simulink model "OCR"  (Simulink 10.0)
settings: Solver=ode23tb  StartTime=0.0  StopTime=10  RelTol=1e-3  EnableMultiTasking=on
libraries: powerlib x36, powerlib_extras x12, simulink x6
settings Model: Creator=Khan  LastModifiedBy=bhisma
settings DataIOCC: LimitDataPoints=on  SignalLoggingSaveFormat=ModelDataLogs
settings OptimizationCC: ExpressionDepthLimit=2147483647  InitFltsAndDblsToZero=on
settings DebuggingCC: SaveWithParameterizedLinksMsg=none  SignalResolutionControl=TryResolveAllWithWarning  MultiTaskDSMMsg=warning  MultiTaskCondExecSysMsg=none  FcnCallInpInsideContextMsg=warning  StateNameClashWarn=warning
settings SFSimCC: SimParseCustomCode=off
settings GRTTargetCC: TargetFcnLib=ansi_tfl_tmw.mat  GeneratePreprocessorConditionals=Disable all
settings ConfigComp: CovExternalEMLEnable=off

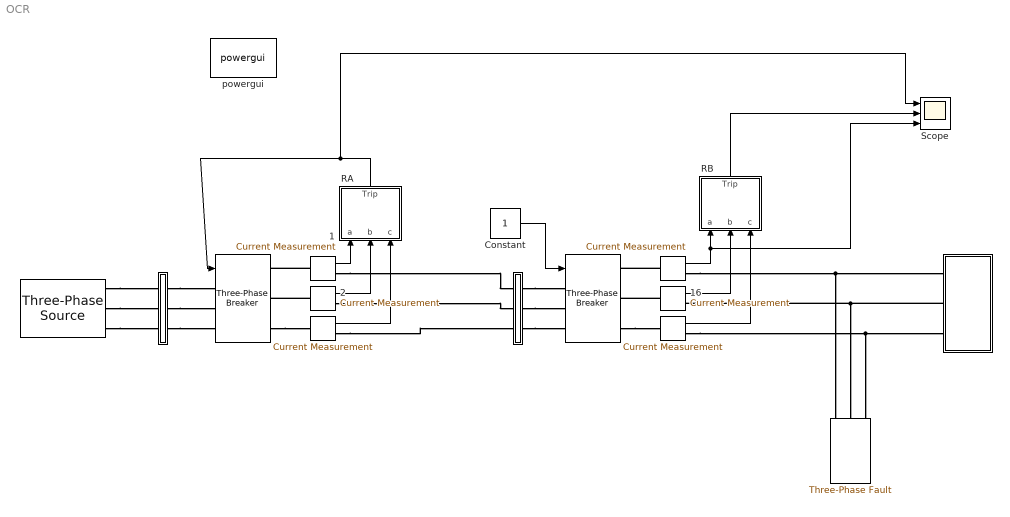
== system OCR ==
  "     " : powerlib/Measurements/Current Measurement  SystemSampleTime=-1  PhasorSimulation=off  OutputType=Complex  PSBequivalent=0
      settings: SourceProductName=Simscape Electrical
  "                                                     " : powerlib/Measurements/Current Measurement  SystemSampleTime=-1  PhasorSimulation=off  OutputType=Complex  PSBequivalent=0
      settings: SourceProductName=Simscape Electrical
  "                                                            " : powerlib/Measurements/Current Measurement  SystemSampleTime=-1  PhasorSimulation=off  OutputType=Complex  PSBequivalent=0
      settings: SourceProductName=Simscape Electrical
  " 1" : powerlib/Measurements/Current Measurement  SystemSampleTime=-1  PhasorSimulation=off  OutputType=Complex  PSBequivalent=0
      settings: SourceProductName=Simscape Electrical
  " 16" : powerlib/Measurements/Current Measurement  SystemSampleTime=-1  PhasorSimulation=off  OutputType=Complex  PSBequivalent=0
      settings: SourceProductName=Simscape Electrical
  " 2" : powerlib/Measurements/Current Measurement  SystemSampleTime=-1  PhasorSimulation=off  OutputType=Complex  PSBequivalent=0
      settings: SourceProductName=Simscape Electrical
  " " : powerlib/Elements/Three-Phase Breaker  SystemSampleTime=-1  InitialState=closed  SwitchA=on  SwitchB=on  SwitchC=on  SwitchTimes=1000000000  External=on  BreakerResistance=0.001  SnubberResistance=1e6  SnubberCapacitance=inf  Measurements=None
      link override Breaker A: Measurements=None
      link override Breaker B: Measurements=None
      link override Breaker C: Measurements=None
      settings: SourceProductName=Simscape Electrical
  "    " : Subsystem
      mask Display: disp('')
  "      " : powerlib/Elements/Three-Phase Breaker  SystemSampleTime=-1  InitialState=closed  SwitchA=on  SwitchB=on  SwitchC=on  SwitchTimes=1000000000  External=on  BreakerResistance=0.001  SnubberResistance=1e6  SnubberCapacitance=inf  Measurements=None
      link override Breaker A: Measurements=None
      link override Breaker B: Measurements=None
      link override Breaker C: Measurements=None
      settings: SourceProductName=Simscape Electrical
  "       " : Subsystem
      mask Display: disp('')
  "               " : powerlib/Elements/Three-Phase Fault  SystemSampleTime=-1  FaultA=on  FaultB=on  FaultC=on  FaultResistance=0.6  GroundFault=on  GroundResistance=1000000  External=off  SwitchStatus=[1]  SwitchTimes=[ 6]  InitialStates=[0 0 1]  SnubberResistance=1e6  SnubberCapacitance=inf  Measurements=None
      settings: SourceProductName=Simscape Electrical
  "                            " : Subsystem
  "                                           " : powerlib/Electrical Sources/Three-Phase Source  SystemSampleTime=-1  Voltage=400  PhaseAngle=0  Frequency=50  InternalConnection=Yg  SpecifyImpedance=on  Resistance=25^2/1000/10  Inductance=25^2/1000/377  ShortCircuitLevel=1020e6  BaseVoltage=400  XRratio=10
      settings: SourceProductName=Simscape Electrical
  Constant : Constant
  RA : Subsystem
  RB : Subsystem
  Scope : Scope  NumInputPorts=3
  powergui : powerlib/powergui  Priority=1  SystemSampleTime=-1  SimulationMode=Continuous  SampleTime=50e-6  frequency=60  SPID=off  DisableSnubberDevices=off  DisableRonSwitches=off  DisableVfSwitches=off  SwTol=0  Interpol=off  frequencyindice=0  echomessages=off  HookPort=off  DisplayEquations=off  FunctionMessages=off  EnableUseOfTLC=off  x0status=blocks  RestoreLinks=warning  ResistiveCurrentMeasurement=off  Ylog=off  Xlog=on  ShowGrid=off  save=off  variable=ZData  ZoomFFT=off  StartTime=0.0  cycles=1  DisplayStyle=1  FreqAxis=off  MaxFrequency=1000  frequencyindicesteady=1  display=off  methode=off
      settings: SourceProductName=Simscape Electrical
  wires:
  "                                                            "/1 -> Scope/3, RB/1(a)
  " 16"/1 -> RB/2(b)
  "                                                     "/1 -> RB/3(c)
  RB/1(Trip) -> Scope/2
  " 1"/1 -> RA/1(a)
  " 2"/1 -> RA/2(b)
  "     "/1 -> RA/3(c)
  RA/1(Trip) -> "      "/1, Scope/1
  Constant/1 -> " "/1
  connections:
  "                                                            "/LConn1 -- " "/RConn1
  " 16"/LConn1 -- " "/RConn2
  " "/RConn3 -- "                                                     "/LConn1
  "                                                            "/RConn1 -- "                            "/LConn1 -- "               "/LConn1
  "                            "/LConn2 -- " 16"/RConn1 -- "               "/LConn2
  "                                                     "/RConn1 -- "                            "/LConn3 -- "               "/LConn3
  " 2"/LConn1 -- "      "/RConn2
  " 1"/LConn1 -- "      "/RConn1
  "      "/RConn3 -- "     "/LConn1
  "    "/RConn3 -- " "/LConn3
  "    "/RConn2 -- " "/LConn2
  "    "/RConn1 -- " "/LConn1
  " 1"/RConn1 -- "    "/LConn1
  " 2"/RConn1 -- "    "/LConn2
  "     "/RConn1 -- "    "/LConn3
  "                                           "/RConn3 -- "       "/RConn3
  "                                           "/RConn2 -- "       "/RConn2
  "                                           "/RConn1 -- "       "/RConn1
  "       "/LConn3 -- "      "/LConn3
  "       "/LConn2 -- "      "/LConn2
  "       "/LConn1 -- "      "/LConn1

== system OCR/     ==
  A1 : PMIOPort  Side=Left
  B1 : PMIOPort  Port=2  Side=Left
  C1 : PMIOPort  Port=3  Side=Left
  A2 : PMIOPort  Port=4  Side=Right
  B2 : PMIOPort  Port=5  Side=Right
  C2 : PMIOPort  Port=6  Side=Right
  connections:
  C1/RConn1 -- C2/RConn1
  B1/RConn1 -- B2/RConn1
  A1/RConn1 -- A2/RConn1

== system OCR/        ==
  A1 : PMIOPort  Side=Left
  B1 : PMIOPort  Port=2  Side=Left
  C1 : PMIOPort  Port=3  Side=Left
  A2 : PMIOPort  Port=4  Side=Right
  B2 : PMIOPort  Port=5  Side=Right
  C2 : PMIOPort  Port=6  Side=Right
  connections:
  A1/RConn1 -- A2/RConn1
  B1/RConn1 -- B2/RConn1
  C1/RConn1 -- C2/RConn1

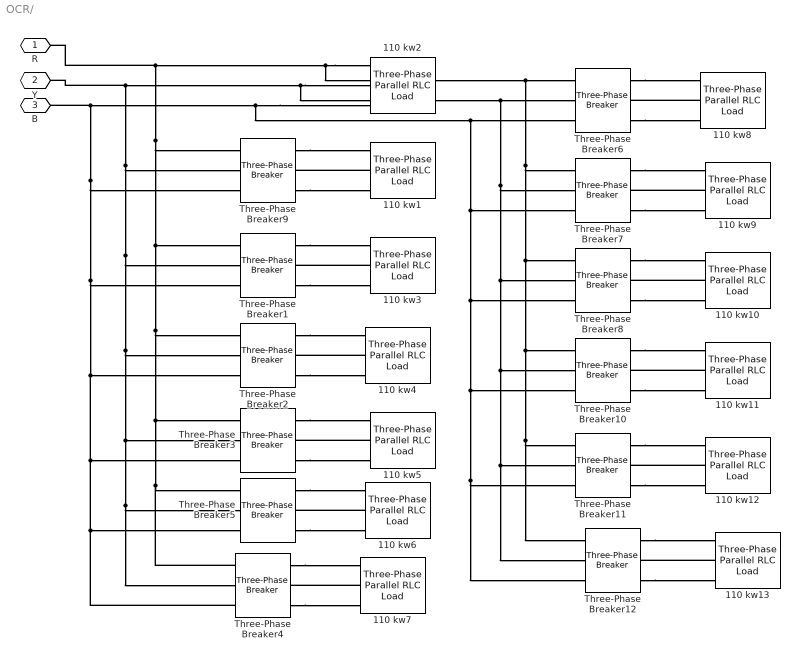
== system OCR/                             ==
  110 kw{1,3..13} (12 alike) : powerlib/Elements/Three-Phase Parallel RLC Load  PhysicalDomain=powersysdomain  SubClassName=unknown  LeftPortType=p1  RightPortType=p1  LConnTagsString=A|B|C  Configuration=Y (grounded)  NominalVoltage=400  NominalFrequency=50  ActivePower=110e3/4  InductivePower=58e3/4  CapacitivePower=0  Measurements=None
      settings: SourceProductName=Simscape Electrical
  110 kw2 : powerlib/Elements/Three-Phase Parallel RLC Load  PhysicalDomain=powersysdomain  SubClassName=unknown  LeftPortType=p1  RightPortType=p1  LConnTagsString=A|B|C  Configuration=Y (grounded)  NominalVoltage=400  NominalFrequency=50  ActivePower=110e3  InductivePower=58e3  CapacitivePower=0  Measurements=None
      settings: SourceProductName=Simscape Electrical
  Three-Phase Breaker1 : powerlib/Elements/Three-Phase Breaker  SystemSampleTime=-1  InitialState=closed  SwitchA=on  SwitchB=on  SwitchC=on  SwitchTimes=1.25  External=off  BreakerResistance=0.001  SnubberResistance=1e6  SnubberCapacitance=inf  Measurements=None
      settings: SourceProductName=Simscape Electrical
  Three-Phase Breaker10 : powerlib/Elements/Three-Phase Breaker  SystemSampleTime=-1  InitialState=closed  SwitchA=on  SwitchB=on  SwitchC=on  SwitchTimes=2.25  External=off  BreakerResistance=0.001  SnubberResistance=1e6  SnubberCapacitance=inf  Measurements=None
      settings: SourceProductName=Simscape Electrical
  Three-Phase Breaker11 : powerlib/Elements/Three-Phase Breaker  SystemSampleTime=-1  InitialState=closed  SwitchA=on  SwitchB=on  SwitchC=on  SwitchTimes=2  External=off  BreakerResistance=0.001  SnubberResistance=1e6  SnubberCapacitance=inf  Measurements=None
      settings: SourceProductName=Simscape Electrical
  Three-Phase Breaker12 : powerlib/Elements/Three-Phase Breaker  SystemSampleTime=-1  InitialState=closed  SwitchA=on  SwitchB=on  SwitchC=on  SwitchTimes=1.75  External=off  BreakerResistance=0.001  SnubberResistance=1e6  SnubberCapacitance=inf  Measurements=None
      settings: SourceProductName=Simscape Electrical
  Three-Phase Breaker2 : powerlib/Elements/Three-Phase Breaker  SystemSampleTime=-1  InitialState=closed  SwitchA=on  SwitchB=on  SwitchC=on  SwitchTimes=1  External=off  BreakerResistance=0.001  SnubberResistance=1e6  SnubberCapacitance=inf  Measurements=None
      settings: SourceProductName=Simscape Electrical
  Three-Phase Breaker3 : powerlib/Elements/Three-Phase Breaker  SystemSampleTime=-1  InitialState=closed  SwitchA=on  SwitchB=on  SwitchC=on  SwitchTimes=0.75  External=off  BreakerResistance=0.001  SnubberResistance=1e6  SnubberCapacitance=inf  Measurements=None
      settings: SourceProductName=Simscape Electrical
  Three-Phase Breaker4 : powerlib/Elements/Three-Phase Breaker  SystemSampleTime=-1  InitialState=closed  SwitchA=on  SwitchB=on  SwitchC=on  SwitchTimes=0.25  External=off  BreakerResistance=0.001  SnubberResistance=1e6  SnubberCapacitance=inf  Measurements=None
      settings: SourceProductName=Simscape Electrical
  Three-Phase Breaker5 : powerlib/Elements/Three-Phase Breaker  SystemSampleTime=-1  InitialState=closed  SwitchA=on  SwitchB=on  SwitchC=on  SwitchTimes=0.5  External=off  BreakerResistance=0.001  SnubberResistance=1e6  SnubberCapacitance=inf  Measurements=None
      settings: SourceProductName=Simscape Electrical
  Three-Phase Breaker6 : powerlib/Elements/Three-Phase Breaker  SystemSampleTime=-1  InitialState=closed  SwitchA=on  SwitchB=on  SwitchC=on  SwitchTimes=3  External=off  BreakerResistance=0.001  SnubberResistance=1e6  SnubberCapacitance=inf  Measurements=None
      settings: SourceProductName=Simscape Electrical
  Three-Phase Breaker7 : powerlib/Elements/Three-Phase Breaker  SystemSampleTime=-1  InitialState=closed  SwitchA=on  SwitchB=on  SwitchC=on  SwitchTimes=2.75  External=off  BreakerResistance=0.001  SnubberResistance=1e6  SnubberCapacitance=inf  Measurements=None
      settings: SourceProductName=Simscape Electrical
  Three-Phase Breaker8 : powerlib/Elements/Three-Phase Breaker  SystemSampleTime=-1  InitialState=closed  SwitchA=on  SwitchB=on  SwitchC=on  SwitchTimes=2.5  External=off  BreakerResistance=0.001  SnubberResistance=1e6  SnubberCapacitance=inf  Measurements=None
      settings: SourceProductName=Simscape Electrical
  Three-Phase Breaker9 : powerlib/Elements/Three-Phase Breaker  SystemSampleTime=-1  InitialState=closed  SwitchA=on  SwitchB=on  SwitchC=on  SwitchTimes=1.5  External=off  BreakerResistance=0.001  SnubberResistance=1e6  SnubberCapacitance=inf  Measurements=None
      settings: SourceProductName=Simscape Electrical
  " R" : PMIOPort  Side=Left
  "Y " : PMIOPort  Port=2  Side=Left
  "B   " : PMIOPort  Port=3  Side=Left
  connections:
  Three-Phase Breaker3/LConn1 -- Three-Phase Breaker4/LConn1 -- Three-Phase Breaker5/LConn1 -- Three-Phase Breaker2/LConn1 -- Three-Phase Breaker1/LConn1 -- Three-Phase Breaker9/LConn1 -- " R"/RConn1 -- 110 kw2/LConn1 -- Three-Phase Breaker6/LConn1 -- Three-Phase Breaker7/LConn1 -- Three-Phase Breaker8/LConn1 -- Three-Phase Breaker10/LConn1 -- Three-Phase Breaker11/LConn1 -- Three-Phase Breaker12/LConn1
  Three-Phase Breaker3/LConn2 -- Three-Phase Breaker4/LConn2 -- Three-Phase Breaker5/LConn2 -- Three-Phase Breaker2/LConn2 -- Three-Phase Breaker1/LConn2 -- Three-Phase Breaker9/LConn2 -- "Y "/RConn1 -- 110 kw2/LConn2 -- Three-Phase Breaker6/LConn2 -- Three-Phase Breaker7/LConn2 -- Three-Phase Breaker8/LConn2 -- Three-Phase Breaker10/LConn2 -- Three-Phase Breaker12/LConn2 -- Three-Phase Breaker11/LConn2
  "B   "/RConn1 -- Three-Phase Breaker12/LConn3 -- Three-Phase Breaker11/LConn3 -- Three-Phase Breaker10/LConn3 -- Three-Phase Breaker8/LConn3 -- Three-Phase Breaker7/LConn3 -- Three-Phase Breaker6/LConn3 -- 110 kw2/LConn3 -- Three-Phase Breaker2/LConn3 -- Three-Phase Breaker3/LConn3 -- Three-Phase Breaker4/LConn3 -- Three-Phase Breaker5/LConn3 -- Three-Phase Breaker1/LConn3 -- Three-Phase Breaker9/LConn3
  Three-Phase Breaker9/RConn1 -- 110 kw1/LConn1
  110 kw1/LConn2 -- Three-Phase Breaker9/RConn2
  Three-Phase Breaker9/RConn3 -- 110 kw1/LConn3
  Three-Phase Breaker1/RConn3 -- 110 kw3/LConn3
  110 kw3/LConn2 -- Three-Phase Breaker1/RConn2
  Three-Phase Breaker1/RConn1 -- 110 kw3/LConn1
  Three-Phase Breaker2/RConn1 -- 110 kw4/LConn1
  110 kw4/LConn2 -- Three-Phase Breaker2/RConn2
  Three-Phase Breaker2/RConn3 -- 110 kw4/LConn3
  Three-Phase Breaker3/RConn3 -- 110 kw5/LConn3
  110 kw5/LConn2 -- Three-Phase Breaker3/RConn2
  Three-Phase Breaker3/RConn1 -- 110 kw5/LConn1
  Three-Phase Breaker4/RConn1 -- 110 kw7/LConn1
  110 kw7/LConn2 -- Three-Phase Breaker4/RConn2
  Three-Phase Breaker4/RConn3 -- 110 kw7/LConn3
  Three-Phase Breaker5/RConn1 -- 110 kw6/LConn1
  110 kw6/LConn2 -- Three-Phase Breaker5/RConn2
  Three-Phase Breaker5/RConn3 -- 110 kw6/LConn3
  Three-Phase Breaker6/RConn3 -- 110 kw8/LConn3
  110 kw8/LConn2 -- Three-Phase Breaker6/RConn2
  Three-Phase Breaker6/RConn1 -- 110 kw8/LConn1
  Three-Phase Breaker7/RConn1 -- 110 kw9/LConn1
  110 kw9/LConn2 -- Three-Phase Breaker7/RConn2
  Three-Phase Breaker7/RConn3 -- 110 kw9/LConn3
  Three-Phase Breaker8/RConn3 -- 110 kw10/LConn3
  Three-Phase Breaker8/RConn1 -- 110 kw10/LConn1
  110 kw10/LConn2 -- Three-Phase Breaker8/RConn2
  110 kw11/LConn2 -- Three-Phase Breaker10/RConn2
  Three-Phase Breaker10/RConn1 -- 110 kw11/LConn1
  Three-Phase Breaker10/RConn3 -- 110 kw11/LConn3
  Three-Phase Breaker11/RConn3 -- 110 kw12/LConn3
  Three-Phase Breaker11/RConn1 -- 110 kw12/LConn1
  110 kw12/LConn2 -- Three-Phase Breaker11/RConn2
  110 kw13/LConn2 -- Three-Phase Breaker12/RConn2
  Three-Phase Breaker12/RConn3 -- 110 kw13/LConn3
  Three-Phase Breaker12/RConn1 -- 110 kw13/LConn1

== system OCR/RA ==
  a : Inport
  b : Inport  Port=2
  c : Inport  Port=3
  " 18" : DataTypeConversion  OutDataTypeStr=double
  Logical Operator : Logic  Inputs=3  AllPortsSameDT=off  OutDataTypeStr=boolean
  phase a : Subsystem
  phase a1 : Subsystem
  phase a2 : Subsystem
  Trip : Outport
  wires:
  " 18"/1 -> Trip/1
  c/1 -> phase a2/1(In1)
  b/1 -> phase a1/1(In1)
  a/1 -> phase a/1(In1)
  phase a/1(Out1) -> Logical Operator/1
  Logical Operator/1 -> " 18"/1
  phase a2/1(Out1) -> Logical Operator/3
  phase a1/1(Out1) -> Logical Operator/2

== system OCR/RB ==
  a : Inport
  b : Inport  Port=2
  c : Inport  Port=3
  " 18" : DataTypeConversion  OutDataTypeStr=double
  Logical Operator : Logic  Inputs=3  AllPortsSameDT=off  OutDataTypeStr=boolean
  phase a : Subsystem
  phase a1 : Subsystem
  phase a2 : Subsystem
  Trip : Outport
  wires:
  phase a1/1(Out1) -> Logical Operator/2
  phase a2/1(Out1) -> Logical Operator/3
  Logical Operator/1 -> " 18"/1
  phase a/1(Out1) -> Logical Operator/1
  a/1 -> phase a/1(In1)
  b/1 -> phase a1/1(In1)
  c/1 -> phase a2/1(In1)
  " 18"/1 -> Trip/1

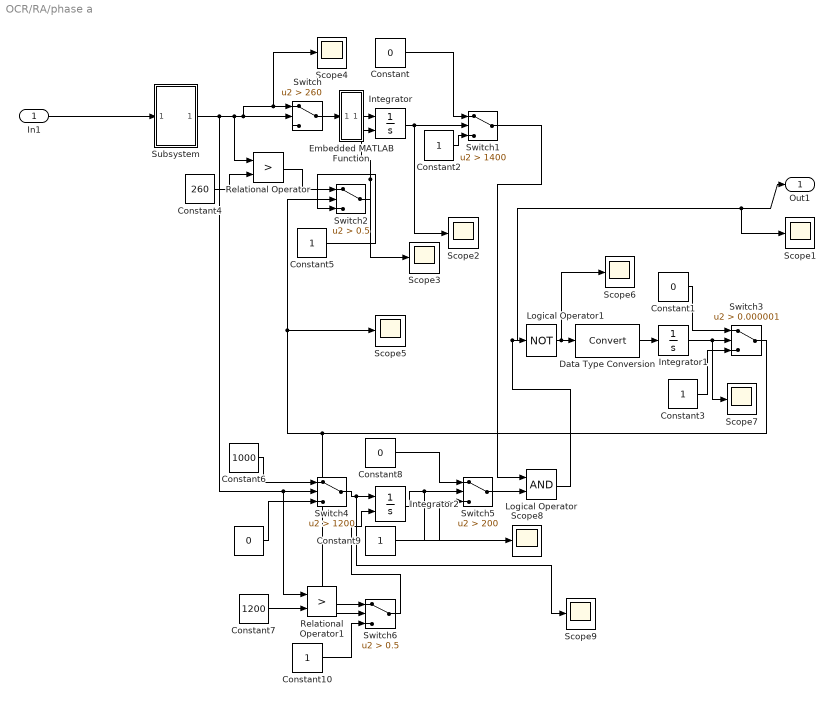
== system OCR/RA/phase a ==
  In1 : Inport
  " " : Constant  Value=0
  Constant : Constant  Value=0
  Constant1 : Constant  Value=0
  Constant{2..3,5,9..10} (5 alike) : Constant
  Constant4 : Constant  Value=260
  Constant6 : Constant  Value=1000
  Constant7 : Constant  Value=1200
  Constant8 : Constant  Value=0
  Data Type Conversion : DataTypeConversion
  Embedded MATLAB Function : MATLAB Function  TreatAsAtomicUnit=on
  Integrator : Integrator  ExternalReset=falling
  Integrator1 : Integrator
  Integrator2 : Integrator  ExternalReset=falling
  Logical Operator : Logic  AllPortsSameDT=off  OutDataTypeStr=boolean
  Logical Operator1 : Logic  Operator=NOT  AllPortsSameDT=off  OutDataTypeStr=boolean
  Relational Operator : RelationalOperator  Operator=>  OutDataTypeStr=boolean  RndMeth=Nearest
  Relational Operator1 : RelationalOperator  Operator=>  OutDataTypeStr=boolean  RndMeth=Nearest
  Scope{1..9} (9 alike) : Scope
  Subsystem : Subsystem
  Switch : Switch  Criteria=u2 > Threshold  Threshold=260
  Switch1 : Switch  Criteria=u2 > Threshold  Threshold=1400  ZeroCross=off
  Switch2 : Switch  Criteria=u2 > Threshold  Threshold=0.5
  Switch3 : Switch  Criteria=u2 > Threshold  Threshold=0.000001
  Switch4 : Switch  Criteria=u2 > Threshold  Threshold=1200
  Switch5 : Switch  Criteria=u2 > Threshold  Threshold=200  ZeroCross=off
  Switch6 : Switch  Criteria=u2 > Threshold  Threshold=0.5
  Out1 : Outport
  wires:
  Switch6/1 -> Integrator2/2
  Constant10/1 -> Switch6/3
  Relational Operator1/1 -> Switch6/1
  Constant7/1 -> Relational Operator1/2
  Logical Operator/1 -> Scope1/1, Out1/1, Logical Operator1/1
  Switch5/1 -> Logical Operator/2
  Constant9/1 -> Switch5/3
  Constant8/1 -> Switch5/1
  Integrator2/1 -> Scope8/1, Switch5/2
  Switch4/1 -> Scope9/1, Integrator2/1
  " "/1 -> Switch4/3
  Constant6/1 -> Switch4/1
  Embedded MATLAB Function/1(y) -> Integrator/1
  Switch3/1 -> Switch6/2, Scope5/1, Switch2/2
  Constant1/1 -> Switch3/1
  Integrator1/1 -> Switch3/2, Scope7/1
  Data Type Conversion/1 -> Integrator1/1
  Logical Operator1/1 -> Data Type Conversion/1, Scope6/1
  Constant2/1 -> Switch1/3
  Switch/1 -> Embedded MATLAB Function/1(u)
  Subsystem/1(Out1) -> Relational Operator1/1, Switch4/2, Scope4/1, Switch/1, Switch/2, Relational Operator/1
  Integrator/1 -> Scope2/1, Switch1/2
  Switch1/1 -> Logical Operator/1
  Constant/1 -> Switch1/1
  In1/1 -> Subsystem/1(In1)
  Constant3/1 -> Switch3/3
  Constant4/1 -> Relational Operator/2
  Relational Operator/1 -> Switch2/1
  Switch2/1 -> Integrator/2, Scope3/1
  Constant5/1 -> Switch2/3

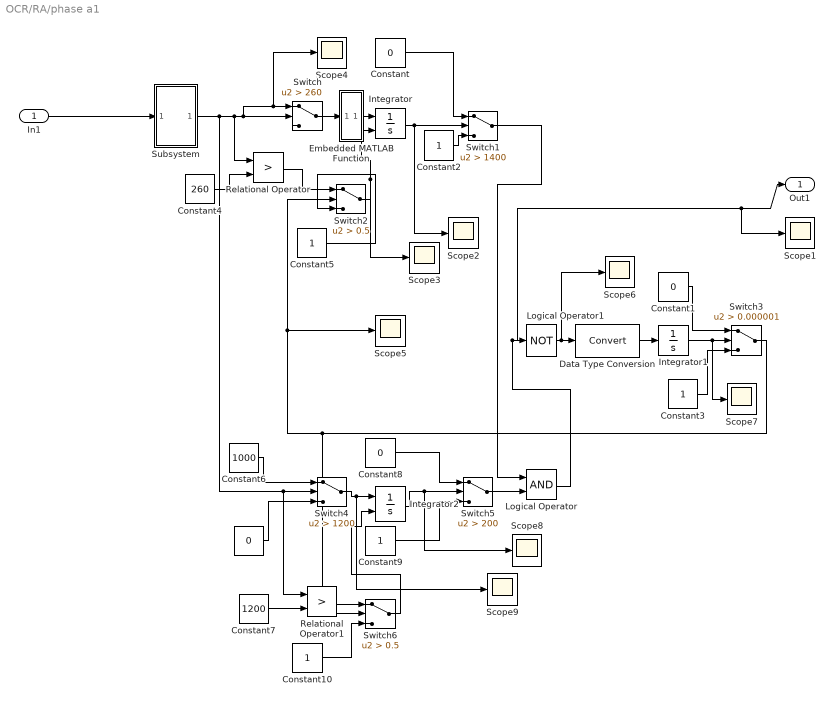
== system OCR/RA/phase a1 ==
  In1 : Inport
  " " : Constant  Value=0
  Constant : Constant  Value=0
  Constant1 : Constant  Value=0
  Constant{2..3,5,9..10} (5 alike) : Constant
  Constant4 : Constant  Value=260
  Constant6 : Constant  Value=1000
  Constant7 : Constant  Value=1200
  Constant8 : Constant  Value=0
  Data Type Conversion : DataTypeConversion
  Embedded MATLAB Function : MATLAB Function  TreatAsAtomicUnit=on
  Integrator : Integrator  ExternalReset=falling
  Integrator1 : Integrator
  Integrator2 : Integrator  ExternalReset=falling
  Logical Operator : Logic  AllPortsSameDT=off  OutDataTypeStr=boolean
  Logical Operator1 : Logic  Operator=NOT  AllPortsSameDT=off  OutDataTypeStr=boolean
  Relational Operator : RelationalOperator  Operator=>  OutDataTypeStr=boolean  RndMeth=Nearest
  Relational Operator1 : RelationalOperator  Operator=>  OutDataTypeStr=boolean  RndMeth=Nearest
  Scope{1..9} (9 alike) : Scope
  Subsystem : Subsystem
  Switch : Switch  Criteria=u2 > Threshold  Threshold=260
  Switch1 : Switch  Criteria=u2 > Threshold  Threshold=1400  ZeroCross=off
  Switch2 : Switch  Criteria=u2 > Threshold  Threshold=0.5
  Switch3 : Switch  Criteria=u2 > Threshold  Threshold=0.000001
  Switch4 : Switch  Criteria=u2 > Threshold  Threshold=1200
  Switch5 : Switch  Criteria=u2 > Threshold  Threshold=200  ZeroCross=off
  Switch6 : Switch  Criteria=u2 > Threshold  Threshold=0.5
  Out1 : Outport
  wires:
  Constant5/1 -> Switch2/3
  Switch2/1 -> Scope3/1, Integrator/2
  Relational Operator/1 -> Switch2/1
  Constant4/1 -> Relational Operator/2
  Constant3/1 -> Switch3/3
  In1/1 -> Subsystem/1(In1)
  Constant/1 -> Switch1/1
  Switch1/1 -> Logical Operator/1
  Integrator/1 -> Switch1/2, Scope2/1
  Subsystem/1(Out1) -> Relational Operator/1, Switch/2, Switch/1, Scope4/1, Switch4/2, Relational Operator1/1
  Switch/1 -> Embedded MATLAB Function/1(u)
  Constant2/1 -> Switch1/3
  Logical Operator1/1 -> Scope6/1, Data Type Conversion/1
  Data Type Conversion/1 -> Integrator1/1
  Integrator1/1 -> Scope7/1, Switch3/2
  Constant1/1 -> Switch3/1
  Switch3/1 -> Switch2/2, Scope5/1, Switch6/2
  Embedded MATLAB Function/1(y) -> Integrator/1
  Constant6/1 -> Switch4/1
  " "/1 -> Switch4/3
  Switch4/1 -> Integrator2/1, Scope9/1
  Integrator2/1 -> Switch5/2, Scope8/1
  Constant8/1 -> Switch5/1
  Constant9/1 -> Switch5/3
  Switch5/1 -> Logical Operator/2
  Logical Operator/1 -> Logical Operator1/1, Out1/1, Scope1/1
  Constant7/1 -> Relational Operator1/2
  Relational Operator1/1 -> Switch6/1
  Constant10/1 -> Switch6/3
  Switch6/1 -> Integrator2/2

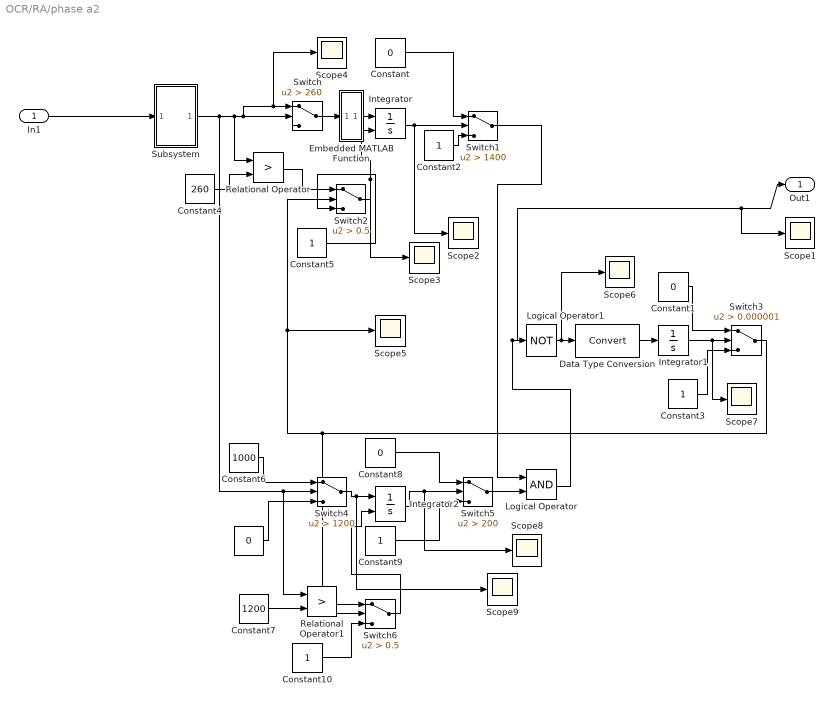
== system OCR/RA/phase a2 ==
  In1 : Inport
  " " : Constant  Value=0
  Constant : Constant  Value=0
  Constant1 : Constant  Value=0
  Constant{2..3,5,9..10} (5 alike) : Constant
  Constant4 : Constant  Value=260
  Constant6 : Constant  Value=1000
  Constant7 : Constant  Value=1200
  Constant8 : Constant  Value=0
  Data Type Conversion : DataTypeConversion
  Embedded MATLAB Function : MATLAB Function  TreatAsAtomicUnit=on
  Integrator : Integrator  ExternalReset=falling
  Integrator1 : Integrator
  Integrator2 : Integrator  ExternalReset=falling
  Logical Operator : Logic  AllPortsSameDT=off  OutDataTypeStr=boolean
  Logical Operator1 : Logic  Operator=NOT  AllPortsSameDT=off  OutDataTypeStr=boolean
  Relational Operator : RelationalOperator  Operator=>  OutDataTypeStr=boolean  RndMeth=Nearest
  Relational Operator1 : RelationalOperator  Operator=>  OutDataTypeStr=boolean  RndMeth=Nearest
  Scope{1..9} (9 alike) : Scope
  Subsystem : Subsystem
  Switch : Switch  Criteria=u2 > Threshold  Threshold=260
  Switch1 : Switch  Criteria=u2 > Threshold  Threshold=1400  ZeroCross=off
  Switch2 : Switch  Criteria=u2 > Threshold  Threshold=0.5
  Switch3 : Switch  Criteria=u2 > Threshold  Threshold=0.000001
  Switch4 : Switch  Criteria=u2 > Threshold  Threshold=1200
  Switch5 : Switch  Criteria=u2 > Threshold  Threshold=200  ZeroCross=off
  Switch6 : Switch  Criteria=u2 > Threshold  Threshold=0.5
  Out1 : Outport
  wires:
  Switch6/1 -> Integrator2/2
  Constant10/1 -> Switch6/3
  Relational Operator1/1 -> Switch6/1
  Constant7/1 -> Relational Operator1/2
  Logical Operator/1 -> Scope1/1, Out1/1, Logical Operator1/1
  Switch5/1 -> Logical Operator/2
  Constant9/1 -> Switch5/3
  Constant8/1 -> Switch5/1
  Integrator2/1 -> Scope8/1, Switch5/2
  Switch4/1 -> Scope9/1, Integrator2/1
  " "/1 -> Switch4/3
  Constant6/1 -> Switch4/1
  Embedded MATLAB Function/1(y) -> Integrator/1
  Switch3/1 -> Switch6/2, Scope5/1, Switch2/2
  Constant1/1 -> Switch3/1
  Integrator1/1 -> Switch3/2, Scope7/1
  Data Type Conversion/1 -> Integrator1/1
  Logical Operator1/1 -> Data Type Conversion/1, Scope6/1
  Constant2/1 -> Switch1/3
  Switch/1 -> Embedded MATLAB Function/1(u)
  Subsystem/1(Out1) -> Relational Operator1/1, Switch4/2, Scope4/1, Switch/1, Switch/2, Relational Operator/1
  Integrator/1 -> Scope2/1, Switch1/2
  Switch1/1 -> Logical Operator/1
  Constant/1 -> Switch1/1
  In1/1 -> Subsystem/1(In1)
  Constant3/1 -> Switch3/3
  Constant4/1 -> Relational Operator/2
  Relational Operator/1 -> Switch2/1
  Switch2/1 -> Integrator/2, Scope3/1
  Constant5/1 -> Switch2/3

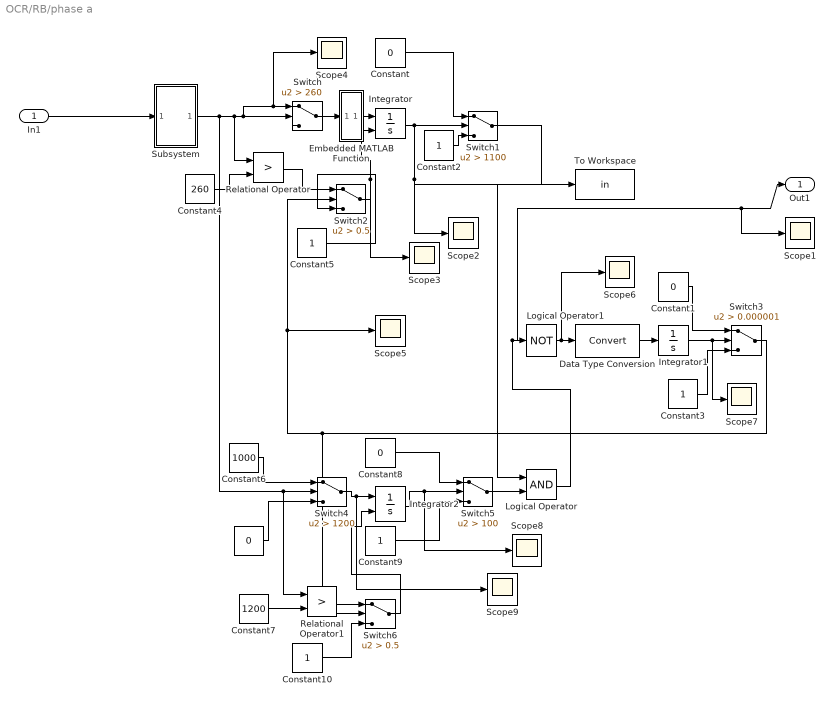
== system OCR/RB/phase a ==
  In1 : Inport
  " " : Constant  Value=0
  Constant : Constant  Value=0
  Constant1 : Constant  Value=0
  Constant{2..3,5,9..10} (5 alike) : Constant
  Constant4 : Constant  Value=260
  Constant6 : Constant  Value=1000
  Constant7 : Constant  Value=1200
  Constant8 : Constant  Value=0
  Data Type Conversion : DataTypeConversion
  Embedded MATLAB Function : MATLAB Function  TreatAsAtomicUnit=on
  Integrator : Integrator  ExternalReset=falling
  Integrator1 : Integrator
  Integrator2 : Integrator  ExternalReset=falling
  Logical Operator : Logic  AllPortsSameDT=off  OutDataTypeStr=boolean
  Logical Operator1 : Logic  Operator=NOT  AllPortsSameDT=off  OutDataTypeStr=boolean
  Relational Operator : RelationalOperator  Operator=>  OutDataTypeStr=boolean  RndMeth=Nearest
  Relational Operator1 : RelationalOperator  Operator=>  OutDataTypeStr=boolean  RndMeth=Nearest
  Scope{1..9} (9 alike) : Scope
  Subsystem : Subsystem
  Switch : Switch  Criteria=u2 > Threshold  Threshold=260
  Switch1 : Switch  Criteria=u2 > Threshold  Threshold=1100  ZeroCross=off
  Switch2 : Switch  Criteria=u2 > Threshold  Threshold=0.5
  Switch3 : Switch  Criteria=u2 > Threshold  Threshold=0.000001
  Switch4 : Switch  Criteria=u2 > Threshold  Threshold=1200
  Switch5 : Switch  Criteria=u2 > Threshold  Threshold=100  ZeroCross=off
  Switch6 : Switch  Criteria=u2 > Threshold  Threshold=0.5
  To Workspace : ToWorkspace  VariableName=in  SampleTime=-1
  Out1 : Outport
  wires:
  Constant5/1 -> Switch2/3
  Switch2/1 -> Scope3/1, Integrator/2
  Relational Operator/1 -> Switch2/1
  Constant4/1 -> Relational Operator/2
  Constant3/1 -> Switch3/3
  In1/1 -> Subsystem/1(In1)
  Constant/1 -> Switch1/1
  Switch1/1 -> Logical Operator/1
  Integrator/1 -> Switch1/2, Scope2/1, To Workspace/1
  Subsystem/1(Out1) -> Relational Operator/1, Switch/2, Switch/1, Scope4/1, Switch4/2, Relational Operator1/1
  Switch/1 -> Embedded MATLAB Function/1(u)
  Constant2/1 -> Switch1/3
  Logical Operator1/1 -> Scope6/1, Data Type Conversion/1
  Data Type Conversion/1 -> Integrator1/1
  Integrator1/1 -> Scope7/1, Switch3/2
  Constant1/1 -> Switch3/1
  Switch3/1 -> Switch2/2, Scope5/1, Switch6/2
  Embedded MATLAB Function/1(y) -> Integrator/1
  Constant6/1 -> Switch4/1
  " "/1 -> Switch4/3
  Switch4/1 -> Integrator2/1, Scope9/1
  Integrator2/1 -> Switch5/2, Scope8/1
  Constant8/1 -> Switch5/1
  Constant9/1 -> Switch5/3
  Switch5/1 -> Logical Operator/2
  Logical Operator/1 -> Logical Operator1/1, Out1/1, Scope1/1
  Constant7/1 -> Relational Operator1/2
  Relational Operator1/1 -> Switch6/1
  Constant10/1 -> Switch6/3
  Switch6/1 -> Integrator2/2

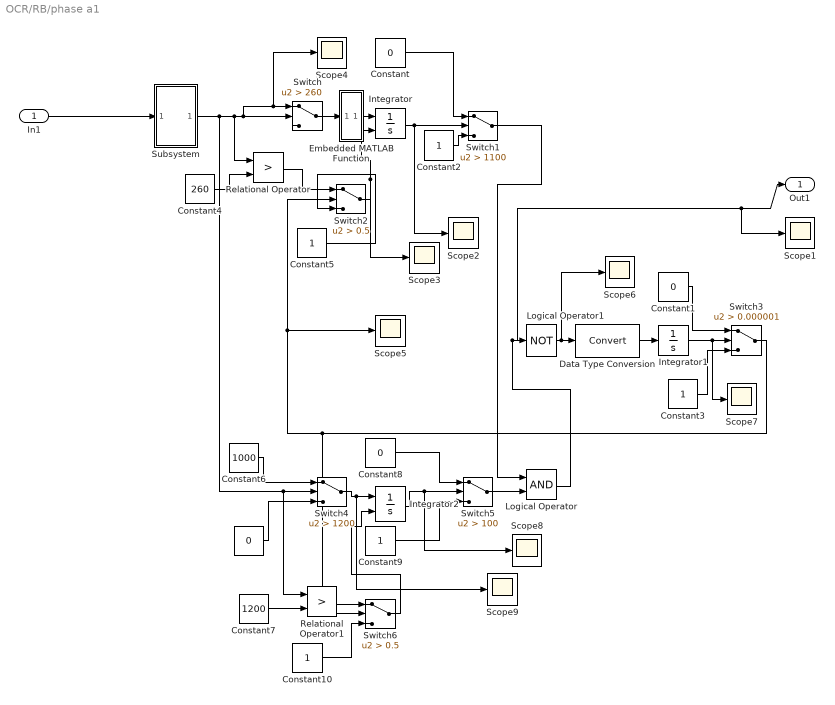
== system OCR/RB/phase a1 ==
  In1 : Inport
  " " : Constant  Value=0
  Constant : Constant  Value=0
  Constant1 : Constant  Value=0
  Constant{2..3,5,9..10} (5 alike) : Constant
  Constant4 : Constant  Value=260
  Constant6 : Constant  Value=1000
  Constant7 : Constant  Value=1200
  Constant8 : Constant  Value=0
  Data Type Conversion : DataTypeConversion
  Embedded MATLAB Function : MATLAB Function  TreatAsAtomicUnit=on
  Integrator : Integrator  ExternalReset=falling
  Integrator1 : Integrator
  Integrator2 : Integrator  ExternalReset=falling
  Logical Operator : Logic  AllPortsSameDT=off  OutDataTypeStr=boolean
  Logical Operator1 : Logic  Operator=NOT  AllPortsSameDT=off  OutDataTypeStr=boolean
  Relational Operator : RelationalOperator  Operator=>  OutDataTypeStr=boolean  RndMeth=Nearest
  Relational Operator1 : RelationalOperator  Operator=>  OutDataTypeStr=boolean  RndMeth=Nearest
  Scope{1..9} (9 alike) : Scope
  Subsystem : Subsystem
  Switch : Switch  Criteria=u2 > Threshold  Threshold=260
  Switch1 : Switch  Criteria=u2 > Threshold  Threshold=1100  ZeroCross=off
  Switch2 : Switch  Criteria=u2 > Threshold  Threshold=0.5
  Switch3 : Switch  Criteria=u2 > Threshold  Threshold=0.000001
  Switch4 : Switch  Criteria=u2 > Threshold  Threshold=1200
  Switch5 : Switch  Criteria=u2 > Threshold  Threshold=100  ZeroCross=off
  Switch6 : Switch  Criteria=u2 > Threshold  Threshold=0.5
  Out1 : Outport
  wires:
  Switch6/1 -> Integrator2/2
  Constant10/1 -> Switch6/3
  Relational Operator1/1 -> Switch6/1
  Constant7/1 -> Relational Operator1/2
  Logical Operator/1 -> Scope1/1, Out1/1, Logical Operator1/1
  Switch5/1 -> Logical Operator/2
  Constant9/1 -> Switch5/3
  Constant8/1 -> Switch5/1
  Integrator2/1 -> Scope8/1, Switch5/2
  Switch4/1 -> Scope9/1, Integrator2/1
  " "/1 -> Switch4/3
  Constant6/1 -> Switch4/1
  Embedded MATLAB Function/1(y) -> Integrator/1
  Switch3/1 -> Switch6/2, Scope5/1, Switch2/2
  Constant1/1 -> Switch3/1
  Integrator1/1 -> Switch3/2, Scope7/1
  Data Type Conversion/1 -> Integrator1/1
  Logical Operator1/1 -> Data Type Conversion/1, Scope6/1
  Constant2/1 -> Switch1/3
  Switch/1 -> Embedded MATLAB Function/1(u)
  Subsystem/1(Out1) -> Relational Operator1/1, Switch4/2, Scope4/1, Switch/1, Switch/2, Relational Operator/1
  Integrator/1 -> Scope2/1, Switch1/2
  Switch1/1 -> Logical Operator/1
  Constant/1 -> Switch1/1
  In1/1 -> Subsystem/1(In1)
  Constant3/1 -> Switch3/3
  Constant4/1 -> Relational Operator/2
  Relational Operator/1 -> Switch2/1
  Switch2/1 -> Integrator/2, Scope3/1
  Constant5/1 -> Switch2/3

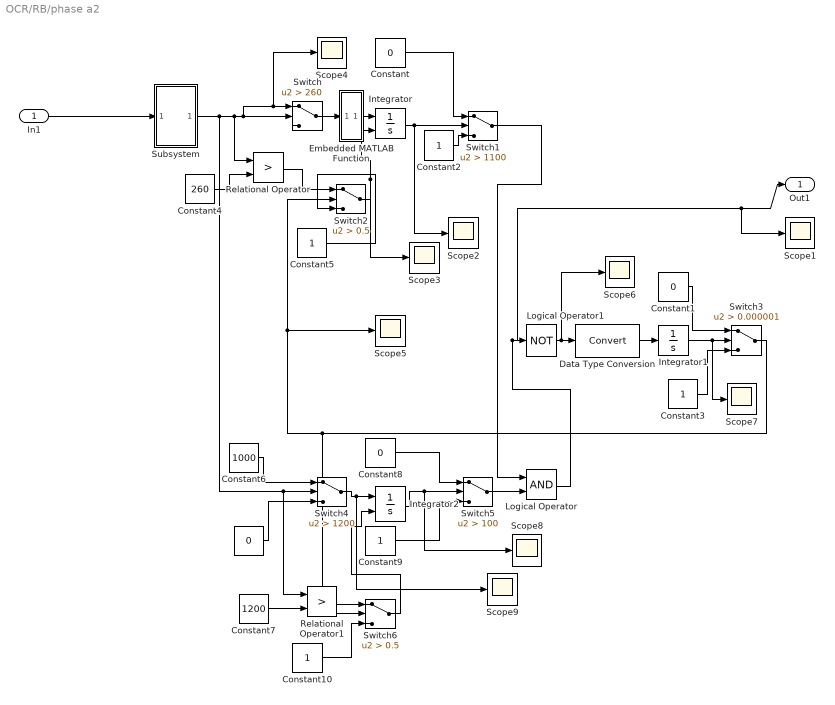
== system OCR/RB/phase a2 ==
  In1 : Inport
  " " : Constant  Value=0
  Constant : Constant  Value=0
  Constant1 : Constant  Value=0
  Constant{2..3,5,9..10} (5 alike) : Constant
  Constant4 : Constant  Value=260
  Constant6 : Constant  Value=1000
  Constant7 : Constant  Value=1200
  Constant8 : Constant  Value=0
  Data Type Conversion : DataTypeConversion
  Embedded MATLAB Function : MATLAB Function  TreatAsAtomicUnit=on
  Integrator : Integrator  ExternalReset=falling
  Integrator1 : Integrator
  Integrator2 : Integrator  ExternalReset=falling
  Logical Operator : Logic  AllPortsSameDT=off  OutDataTypeStr=boolean
  Logical Operator1 : Logic  Operator=NOT  AllPortsSameDT=off  OutDataTypeStr=boolean
  Relational Operator : RelationalOperator  Operator=>  OutDataTypeStr=boolean  RndMeth=Nearest
  Relational Operator1 : RelationalOperator  Operator=>  OutDataTypeStr=boolean  RndMeth=Nearest
  Scope{1..9} (9 alike) : Scope
  Subsystem : Subsystem
  Switch : Switch  Criteria=u2 > Threshold  Threshold=260
  Switch1 : Switch  Criteria=u2 > Threshold  Threshold=1100  ZeroCross=off
  Switch2 : Switch  Criteria=u2 > Threshold  Threshold=0.5
  Switch3 : Switch  Criteria=u2 > Threshold  Threshold=0.000001
  Switch4 : Switch  Criteria=u2 > Threshold  Threshold=1200
  Switch5 : Switch  Criteria=u2 > Threshold  Threshold=100  ZeroCross=off
  Switch6 : Switch  Criteria=u2 > Threshold  Threshold=0.5
  Out1 : Outport
  wires:
  Constant5/1 -> Switch2/3
  Switch2/1 -> Scope3/1, Integrator/2
  Relational Operator/1 -> Switch2/1
  Constant4/1 -> Relational Operator/2
  Constant3/1 -> Switch3/3
  In1/1 -> Subsystem/1(In1)
  Constant/1 -> Switch1/1
  Switch1/1 -> Logical Operator/1
  Integrator/1 -> Switch1/2, Scope2/1
  Subsystem/1(Out1) -> Relational Operator/1, Switch/2, Switch/1, Scope4/1, Switch4/2, Relational Operator1/1
  Switch/1 -> Embedded MATLAB Function/1(u)
  Constant2/1 -> Switch1/3
  Logical Operator1/1 -> Scope6/1, Data Type Conversion/1
  Data Type Conversion/1 -> Integrator1/1
  Integrator1/1 -> Scope7/1, Switch3/2
  Constant1/1 -> Switch3/1
  Switch3/1 -> Switch2/2, Scope5/1, Switch6/2
  Embedded MATLAB Function/1(y) -> Integrator/1
  Constant6/1 -> Switch4/1
  " "/1 -> Switch4/3
  Switch4/1 -> Integrator2/1, Scope9/1
  Integrator2/1 -> Switch5/2, Scope8/1
  Constant8/1 -> Switch5/1
  Constant9/1 -> Switch5/3
  Switch5/1 -> Logical Operator/2
  Logical Operator/1 -> Logical Operator1/1, Out1/1, Scope1/1
  Constant7/1 -> Relational Operator1/2
  Relational Operator1/1 -> Switch6/1
  Constant10/1 -> Switch6/3
  Switch6/1 -> Integrator2/2

== system OCR/RA/phase a/Subsystem ==
  In1 : Inport
  Absolute : MATLABFcn  MATLABFcn=abs
  Check zero  Crossing : HitCross
  Derivative : Derivative
  Divide : Product  Inputs=/*
  Gain : Gain  Gain=2*pi
  Hold derivative  till next zero crossing : powerlib_extras/Discrete  Control Blocks/Discrete Sample & Hold  SystemSampleTime=-1  ic=0  Ts=-1
      settings: SourceProductName=Simscape Electrical  SourceProductBaseCode=PS
  "frequency measuremant " : Subsystem
  Out1 : Outport
  wires:
  Divide/1 -> Out1/1
  In1/1 -> Derivative/1, Check zero  Crossing/1, "frequency measuremant "/1(signal)
  Absolute/1 -> Divide/2
  Gain/1 -> Divide/1
  "frequency measuremant "/1("Freq ") -> Gain/1
  Hold derivative  till next zero crossing/1 -> Absolute/1
  Check zero  Crossing/1 -> Hold derivative  till next zero crossing/2
  Derivative/1 -> Hold derivative  till next zero crossing/1

== system OCR/RA/phase a1/Subsystem ==
  In1 : Inport
  Absolute : MATLABFcn  MATLABFcn=abs
  Check zero  Crossing : HitCross
  Derivative : Derivative
  Divide : Product  Inputs=/*
  Gain : Gain  Gain=2*pi
  Hold derivative  till next zero crossing : powerlib_extras/Discrete  Control Blocks/Discrete Sample & Hold  SystemSampleTime=-1  ic=0  Ts=-1
      settings: SourceProductName=Simscape Electrical  SourceProductBaseCode=PS
  "frequency measuremant " : Subsystem
  Out1 : Outport
  wires:
  Derivative/1 -> Hold derivative  till next zero crossing/1
  Check zero  Crossing/1 -> Hold derivative  till next zero crossing/2
  Hold derivative  till next zero crossing/1 -> Absolute/1
  "frequency measuremant "/1("Freq ") -> Gain/1
  Gain/1 -> Divide/1
  Absolute/1 -> Divide/2
  In1/1 -> "frequency measuremant "/1(signal), Check zero  Crossing/1, Derivative/1
  Divide/1 -> Out1/1

== system OCR/RA/phase a2/Subsystem ==
  In1 : Inport
  Absolute : MATLABFcn  MATLABFcn=abs
  Check zero  Crossing : HitCross
  Derivative : Derivative
  Divide : Product  Inputs=/*
  Gain : Gain  Gain=2*pi
  Hold derivative  till next zero crossing : powerlib_extras/Discrete  Control Blocks/Discrete Sample & Hold  SystemSampleTime=-1  ic=0  Ts=-1
      settings: SourceProductName=Simscape Electrical  SourceProductBaseCode=PS
  "frequency measuremant " : Subsystem
  Out1 : Outport
  wires:
  Divide/1 -> Out1/1
  In1/1 -> Derivative/1, Check zero  Crossing/1, "frequency measuremant "/1(signal)
  Absolute/1 -> Divide/2
  Gain/1 -> Divide/1
  "frequency measuremant "/1("Freq ") -> Gain/1
  Hold derivative  till next zero crossing/1 -> Absolute/1
  Check zero  Crossing/1 -> Hold derivative  till next zero crossing/2
  Derivative/1 -> Hold derivative  till next zero crossing/1

== system OCR/RB/phase a/Subsystem ==
  In1 : Inport
  Absolute : MATLABFcn  MATLABFcn=abs
  Check zero  Crossing : HitCross
  Derivative : Derivative
  Divide : Product  Inputs=/*
  Gain : Gain  Gain=2*pi
  Hold derivative  till next zero crossing : powerlib_extras/Discrete  Control Blocks/Discrete Sample & Hold  SystemSampleTime=-1  ic=0  Ts=-1
      settings: SourceProductName=Simscape Electrical  SourceProductBaseCode=PS
  "frequency measuremant " : Subsystem
  Out1 : Outport
  wires:
  Derivative/1 -> Hold derivative  till next zero crossing/1
  Check zero  Crossing/1 -> Hold derivative  till next zero crossing/2
  Hold derivative  till next zero crossing/1 -> Absolute/1
  "frequency measuremant "/1("Freq ") -> Gain/1
  Gain/1 -> Divide/1
  Absolute/1 -> Divide/2
  In1/1 -> "frequency measuremant "/1(signal), Check zero  Crossing/1, Derivative/1
  Divide/1 -> Out1/1

== system OCR/RB/phase a1/Subsystem ==
  In1 : Inport
  Absolute : MATLABFcn  MATLABFcn=abs
  Check zero  Crossing : HitCross
  Derivative : Derivative
  Divide : Product  Inputs=/*
  Gain : Gain  Gain=2*pi
  Hold derivative  till next zero crossing : powerlib_extras/Discrete  Control Blocks/Discrete Sample & Hold  SystemSampleTime=-1  ic=0  Ts=-1
      settings: SourceProductName=Simscape Electrical  SourceProductBaseCode=PS
  "frequency measuremant " : Subsystem
  Out1 : Outport
  wires:
  Divide/1 -> Out1/1
  In1/1 -> Derivative/1, Check zero  Crossing/1, "frequency measuremant "/1(signal)
  Absolute/1 -> Divide/2
  Gain/1 -> Divide/1
  "frequency measuremant "/1("Freq ") -> Gain/1
  Hold derivative  till next zero crossing/1 -> Absolute/1
  Check zero  Crossing/1 -> Hold derivative  till next zero crossing/2
  Derivative/1 -> Hold derivative  till next zero crossing/1

== system OCR/RB/phase a2/Subsystem ==
  In1 : Inport
  Absolute : MATLABFcn  MATLABFcn=abs
  Check zero  Crossing : HitCross
  Derivative : Derivative
  Divide : Product  Inputs=/*
  Gain : Gain  Gain=2*pi
  Hold derivative  till next zero crossing : powerlib_extras/Discrete  Control Blocks/Discrete Sample & Hold  SystemSampleTime=-1  ic=0  Ts=-1
      settings: SourceProductName=Simscape Electrical  SourceProductBaseCode=PS
  "frequency measuremant " : Subsystem
  Out1 : Outport
  wires:
  Derivative/1 -> Hold derivative  till next zero crossing/1
  Check zero  Crossing/1 -> Hold derivative  till next zero crossing/2
  Hold derivative  till next zero crossing/1 -> Absolute/1
  "frequency measuremant "/1("Freq ") -> Gain/1
  Gain/1 -> Divide/1
  Absolute/1 -> Divide/2
  In1/1 -> "frequency measuremant "/1(signal), Check zero  Crossing/1, Derivative/1
  Divide/1 -> Out1/1

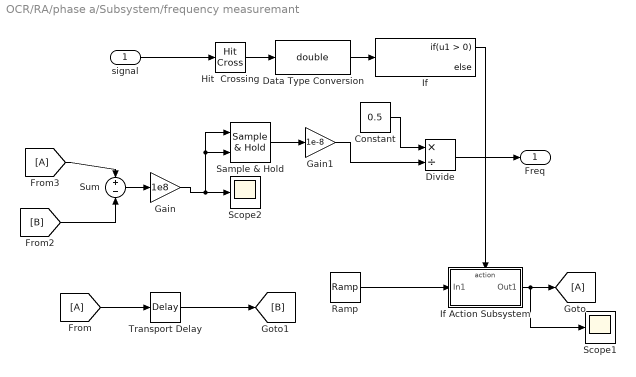
== system OCR/RA/phase a/Subsystem/frequency measuremant  ==
  signal : Inport
  Constant : Constant  Value=0.5
  Data Type Conversion : DataTypeConversion  OutDataTypeStr=double
  Divide : Product  Inputs=*/
  Gain : Gain  Gain=1e8
  Gain1 : Gain  Gain=1e-8
  Hit  Crossing : HitCross
  If : If
  If Action Subsystem : Subsystem  TreatAsAtomicUnit=on
  Ramp : simulink/Sources/Ramp  SystemSampleTime=-1  slope=1  start=0  X0=0
  Sample & Hold : powerlib_extras/Control  Blocks/Sample & Hold  SystemSampleTime=-1  ic=0
      settings: SourceProductName=Simscape Electrical  SourceProductBaseCode=PS
  Scope1 : Scope
  Scope2 : Scope
  Sum : Sum  Inputs=+-
  Transport Delay : TransportDelay  DelayTime=0.0000000000000000000000001
  "Freq " : Outport
  wires:
  Hit  Crossing/1 -> Data Type Conversion/1
  If/1 -> If Action Subsystem/Action
  Ramp/1 -> If Action Subsystem/1(In1)
  If Action Subsystem/1(Out1) -> [A], Scope1/1
  [A] -> Transport Delay/1
  Transport Delay/1 -> [B]
  Data Type Conversion/1 -> If/1
  [A] -> Sum/1
  Sum/1 -> Gain/1
  Sample & Hold/1 -> Gain1/1
  Gain/1 -> Scope2/1, Sample & Hold/1, Sample & Hold/2
  [B] -> Sum/2
  Constant/1 -> Divide/1
  Gain1/1 -> Divide/2
  signal/1 -> Hit  Crossing/1
  Divide/1 -> "Freq "/1

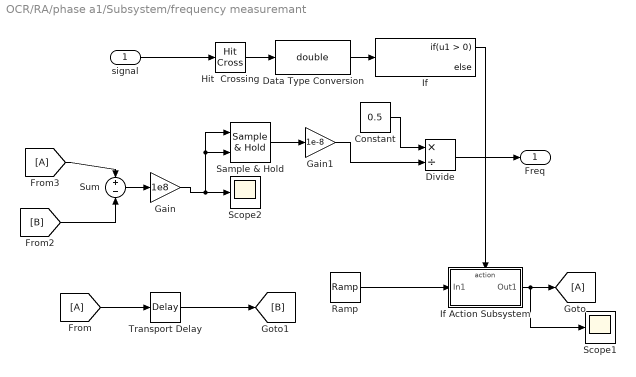
== system OCR/RA/phase a1/Subsystem/frequency measuremant  ==
  signal : Inport
  Constant : Constant  Value=0.5
  Data Type Conversion : DataTypeConversion  OutDataTypeStr=double
  Divide : Product  Inputs=*/
  Gain : Gain  Gain=1e8
  Gain1 : Gain  Gain=1e-8
  Hit  Crossing : HitCross
  If : If
  If Action Subsystem : Subsystem  TreatAsAtomicUnit=on
  Ramp : simulink/Sources/Ramp  SystemSampleTime=-1  slope=1  start=0  X0=0
  Sample & Hold : powerlib_extras/Control  Blocks/Sample & Hold  SystemSampleTime=-1  ic=0
      settings: SourceProductName=Simscape Electrical  SourceProductBaseCode=PS
  Scope1 : Scope
  Scope2 : Scope
  Sum : Sum  Inputs=+-
  Transport Delay : TransportDelay  DelayTime=0.0000000000000000000000001
  "Freq " : Outport
  wires:
  Divide/1 -> "Freq "/1
  signal/1 -> Hit  Crossing/1
  Gain1/1 -> Divide/2
  Constant/1 -> Divide/1
  [B] -> Sum/2
  Gain/1 -> Sample & Hold/2, Sample & Hold/1, Scope2/1
  Sample & Hold/1 -> Gain1/1
  Sum/1 -> Gain/1
  [A] -> Sum/1
  Data Type Conversion/1 -> If/1
  Transport Delay/1 -> [B]
  [A] -> Transport Delay/1
  If Action Subsystem/1(Out1) -> Scope1/1, [A]
  Ramp/1 -> If Action Subsystem/1(In1)
  If/1 -> If Action Subsystem/Action
  Hit  Crossing/1 -> Data Type Conversion/1

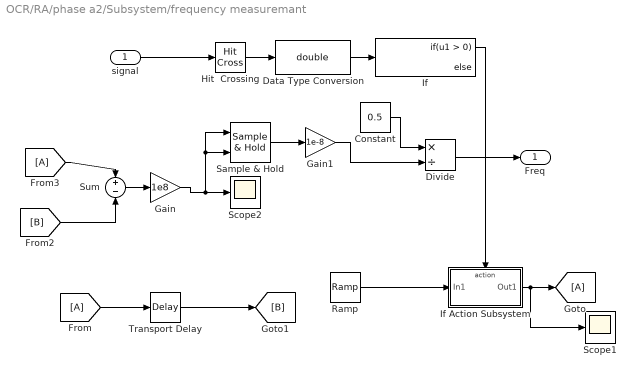
== system OCR/RA/phase a2/Subsystem/frequency measuremant  ==
  signal : Inport
  Constant : Constant  Value=0.5
  Data Type Conversion : DataTypeConversion  OutDataTypeStr=double
  Divide : Product  Inputs=*/
  Gain : Gain  Gain=1e8
  Gain1 : Gain  Gain=1e-8
  Hit  Crossing : HitCross
  If : If
  If Action Subsystem : Subsystem  TreatAsAtomicUnit=on
  Ramp : simulink/Sources/Ramp  SystemSampleTime=-1  slope=1  start=0  X0=0
  Sample & Hold : powerlib_extras/Control  Blocks/Sample & Hold  SystemSampleTime=-1  ic=0
      settings: SourceProductName=Simscape Electrical  SourceProductBaseCode=PS
  Scope1 : Scope
  Scope2 : Scope
  Sum : Sum  Inputs=+-
  Transport Delay : TransportDelay  DelayTime=0.0000000000000000000000001
  "Freq " : Outport
  wires:
  Hit  Crossing/1 -> Data Type Conversion/1
  If/1 -> If Action Subsystem/Action
  Ramp/1 -> If Action Subsystem/1(In1)
  If Action Subsystem/1(Out1) -> [A], Scope1/1
  [A] -> Transport Delay/1
  Transport Delay/1 -> [B]
  Data Type Conversion/1 -> If/1
  [A] -> Sum/1
  Sum/1 -> Gain/1
  Sample & Hold/1 -> Gain1/1
  Gain/1 -> Scope2/1, Sample & Hold/1, Sample & Hold/2
  [B] -> Sum/2
  Constant/1 -> Divide/1
  Gain1/1 -> Divide/2
  signal/1 -> Hit  Crossing/1
  Divide/1 -> "Freq "/1

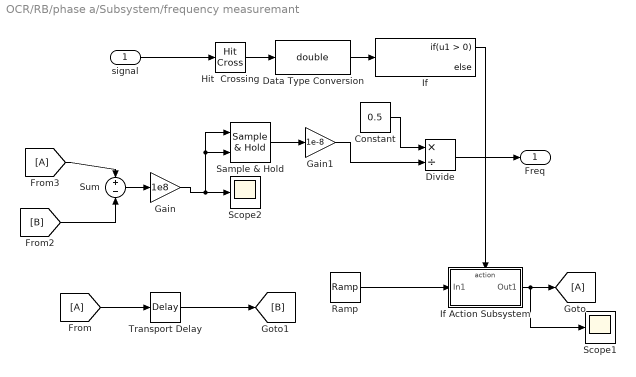
== system OCR/RB/phase a/Subsystem/frequency measuremant  ==
  signal : Inport
  Constant : Constant  Value=0.5
  Data Type Conversion : DataTypeConversion  OutDataTypeStr=double
  Divide : Product  Inputs=*/
  Gain : Gain  Gain=1e8
  Gain1 : Gain  Gain=1e-8
  Hit  Crossing : HitCross
  If : If
  If Action Subsystem : Subsystem  TreatAsAtomicUnit=on
  Ramp : simulink/Sources/Ramp  SystemSampleTime=-1  slope=1  start=0  X0=0
  Sample & Hold : powerlib_extras/Control  Blocks/Sample & Hold  SystemSampleTime=-1  ic=0
      settings: SourceProductName=Simscape Electrical  SourceProductBaseCode=PS
  Scope1 : Scope
  Scope2 : Scope
  Sum : Sum  Inputs=+-
  Transport Delay : TransportDelay  DelayTime=0.0000000000000000000000001
  "Freq " : Outport
  wires:
  Divide/1 -> "Freq "/1
  signal/1 -> Hit  Crossing/1
  Gain1/1 -> Divide/2
  Constant/1 -> Divide/1
  [B] -> Sum/2
  Gain/1 -> Sample & Hold/2, Sample & Hold/1, Scope2/1
  Sample & Hold/1 -> Gain1/1
  Sum/1 -> Gain/1
  [A] -> Sum/1
  Data Type Conversion/1 -> If/1
  Transport Delay/1 -> [B]
  [A] -> Transport Delay/1
  If Action Subsystem/1(Out1) -> Scope1/1, [A]
  Ramp/1 -> If Action Subsystem/1(In1)
  If/1 -> If Action Subsystem/Action
  Hit  Crossing/1 -> Data Type Conversion/1

== system OCR/RB/phase a1/Subsystem/frequency measuremant  ==
  signal : Inport
  Constant : Constant  Value=0.5
  Data Type Conversion : DataTypeConversion  OutDataTypeStr=double
  Divide : Product  Inputs=*/
  Gain : Gain  Gain=1e8
  Gain1 : Gain  Gain=1e-8
  Hit  Crossing : HitCross
  If : If
  If Action Subsystem : Subsystem  TreatAsAtomicUnit=on
  Ramp : simulink/Sources/Ramp  SystemSampleTime=-1  slope=1  start=0  X0=0
  Sample & Hold : powerlib_extras/Control  Blocks/Sample & Hold  SystemSampleTime=-1  ic=0
      settings: SourceProductName=Simscape Electrical  SourceProductBaseCode=PS
  Scope1 : Scope
  Scope2 : Scope
  Sum : Sum  Inputs=+-
  Transport Delay : TransportDelay  DelayTime=0.0000000000000000000000001
  "Freq " : Outport
  wires:
  Hit  Crossing/1 -> Data Type Conversion/1
  If/1 -> If Action Subsystem/Action
  Ramp/1 -> If Action Subsystem/1(In1)
  If Action Subsystem/1(Out1) -> [A], Scope1/1
  [A] -> Transport Delay/1
  Transport Delay/1 -> [B]
  Data Type Conversion/1 -> If/1
  [A] -> Sum/1
  Sum/1 -> Gain/1
  Sample & Hold/1 -> Gain1/1
  Gain/1 -> Scope2/1, Sample & Hold/1, Sample & Hold/2
  [B] -> Sum/2
  Constant/1 -> Divide/1
  Gain1/1 -> Divide/2
  signal/1 -> Hit  Crossing/1
  Divide/1 -> "Freq "/1

== system OCR/RB/phase a2/Subsystem/frequency measuremant  ==
  signal : Inport
  Constant : Constant  Value=0.5
  Data Type Conversion : DataTypeConversion  OutDataTypeStr=double
  Divide : Product  Inputs=*/
  Gain : Gain  Gain=1e8
  Gain1 : Gain  Gain=1e-8
  Hit  Crossing : HitCross
  If : If
  If Action Subsystem : Subsystem  TreatAsAtomicUnit=on
  Ramp : simulink/Sources/Ramp  SystemSampleTime=-1  slope=1  start=0  X0=0
  Sample & Hold : powerlib_extras/Control  Blocks/Sample & Hold  SystemSampleTime=-1  ic=0
      settings: SourceProductName=Simscape Electrical  SourceProductBaseCode=PS
  Scope1 : Scope
  Scope2 : Scope
  Sum : Sum  Inputs=+-
  Transport Delay : TransportDelay  DelayTime=0.0000000000000000000000001
  "Freq " : Outport
  wires:
  Divide/1 -> "Freq "/1
  signal/1 -> Hit  Crossing/1
  Gain1/1 -> Divide/2
  Constant/1 -> Divide/1
  [B] -> Sum/2
  Gain/1 -> Sample & Hold/2, Sample & Hold/1, Scope2/1
  Sample & Hold/1 -> Gain1/1
  Sum/1 -> Gain/1
  [A] -> Sum/1
  Data Type Conversion/1 -> If/1
  Transport Delay/1 -> [B]
  [A] -> Transport Delay/1
  If Action Subsystem/1(Out1) -> Scope1/1, [A]
  Ramp/1 -> If Action Subsystem/1(In1)
  If/1 -> If Action Subsystem/Action
  Hit  Crossing/1 -> Data Type Conversion/1

== system OCR/RA/phase a/Subsystem/frequency measuremant /If Action Subsystem ==
  In1 : Inport
  Action Port : ActionPort  ActionPortLabel=if { }
  Out1 : Outport
  wires:
  In1/1 -> Out1/1

== system OCR/RA/phase a1/Subsystem/frequency measuremant /If Action Subsystem ==
  In1 : Inport
  Action Port : ActionPort  ActionPortLabel=if { }
  Out1 : Outport
  wires:
  In1/1 -> Out1/1

== system OCR/RA/phase a2/Subsystem/frequency measuremant /If Action Subsystem ==
  In1 : Inport
  Action Port : ActionPort  ActionPortLabel=if { }
  Out1 : Outport
  wires:
  In1/1 -> Out1/1

== system OCR/RB/phase a/Subsystem/frequency measuremant /If Action Subsystem ==
  In1 : Inport
  Action Port : ActionPort  ActionPortLabel=if { }
  Out1 : Outport
  wires:
  In1/1 -> Out1/1

== system OCR/RB/phase a1/Subsystem/frequency measuremant /If Action Subsystem ==
  In1 : Inport
  Action Port : ActionPort  ActionPortLabel=if { }
  Out1 : Outport
  wires:
  In1/1 -> Out1/1

== system OCR/RB/phase a2/Subsystem/frequency measuremant /If Action Subsystem ==
  In1 : Inport
  Action Port : ActionPort  ActionPortLabel=if { }
  Out1 : Outport
  wires:
  In1/1 -> Out1/1

== matlab function RA/phase a/Embedded MATLAB Function ==
  data: u input double; y output double
function y = raise_power(u)
%#eml

y = u^0.9;

== matlab function RA/phase a1/Embedded MATLAB Function ==
  data: u input double; y output double
function y = raise_power(u)
%#eml

y = u^0.9;

== matlab function RA/phase a2/Embedded MATLAB Function ==
  data: u input double; y output double
function y = raise_power(u)
%#eml

y = u^0.9;

== matlab function RB/phase a/Embedded MATLAB Function ==
  data: u input double; y output double
function y = raise_power(u)
%#eml

y = u^0.9;

== matlab function RB/phase a1/Embedded MATLAB Function ==
  data: u input double; y output double
function y = raise_power(u)
%#eml

y = u^0.9;

== matlab function RB/phase a2/Embedded MATLAB Function ==
  data: u input double; y output double
function y = raise_power(u)
%#eml

y = u^0.9;
